simulink model "udptest"  (R2017a)
settings: Solver=VariableStepAuto  StartTime=0.0  StopTime=inf  RelTol=1e-3
libraries: ptplib x1, instrumentlib x1, dspnetwork x1
settings Model: xpc_rtwmakecfg_data=_xpciplib__xpcetherlib__xpcether8255xlib__xpcetherGbElib__xpcnblib_  Creator=Barti  LastModifiedBy=Barti

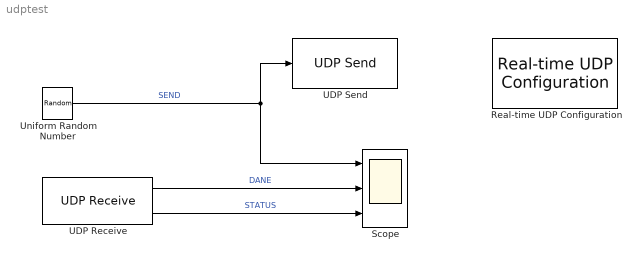
== system udptest ==
  "Real-time UDP Configuration " : ptplib/PTP UDP/Real-time UDP  Configuration   ID=1  IpAddress=192.168.0.10  SubnetMask=255.255.255.0  Gateway=0.0.0.0  EthDrv=Intel 8255x  PciBus=5  PciSlot=0  udpID=0  MulticastList=[]  Multicast={}
      settings: SourceProductName=Simulink Real-Time  SourceProductBaseCode=XP
  Scope : Scope  NumInputPorts=3
  UDP Receive : instrumentlib/UDP Receive  Host=192.168.0.15  Port=8889  LocalPort=22000  DataSize=2  EnableBlockingMode=off  Timeout=10  SampleTime=0.01  DataType=int32  ByteOrder=LittleEndian
      settings: SourceProductName=Instrument Control Toolbox
  UDP Send : dspnetwork/UDP Send  remoteURL='192.168.0.15'  remotePort=8889  localURL='0.0.0.0'  localPortSource=Specify via dialog  localPort=22001  sampletime=-1  blockPlatform=[]  separateLengthPort=0
  Uniform Random Number : UniformRandomNumber  Minimum=2000  Maximum=3000  SampleTime=2
  wires:
  UDP Receive/2 -> Scope/3  "STATUS"
  Uniform Random Number/1 -> Scope/1, UDP Send/1  "SEND"
  UDP Receive/1 -> Scope/2  "DANE"
